simulink model "automode_simple"  (R2020b)
settings: Solver=VariableStepAuto  StartTime=0.0  StopTime=0.1  FixedStep=0.001  RelTol=1e-3
InitFcn:
  | Lf = 0.6*10^-3;
  | Cf = 1338 * 10^-6;
  | Rf = 0.019;
  | f_ac = 60;
  | f_sample = 20*10^3;
  | 
  | R_f = 19e-3;
  | L_f = 0.6e-3;
  | C_f = 1338e-6;
  | RL=2;
  | 
  | A = [0 1/C_f; -1/L_f -R_f/L_f];
  | B = [0 -1/C_f; 1/L_f 0];
  | C = [1 0; 1/RL 0; 0 1];
  | D = zeros(3,2);
libraries: fl_lib x22, nesl_utility x18, ee_lib x15, simulink x4, powerlib_meascontrol x1
settings Model: Creator=Kerim  LastModifiedBy=Kerim
settings SolverCC: ZeroCrossAlgorithm=Adaptive
settings DebuggingCC: IgnoredZcDiagnostic=none

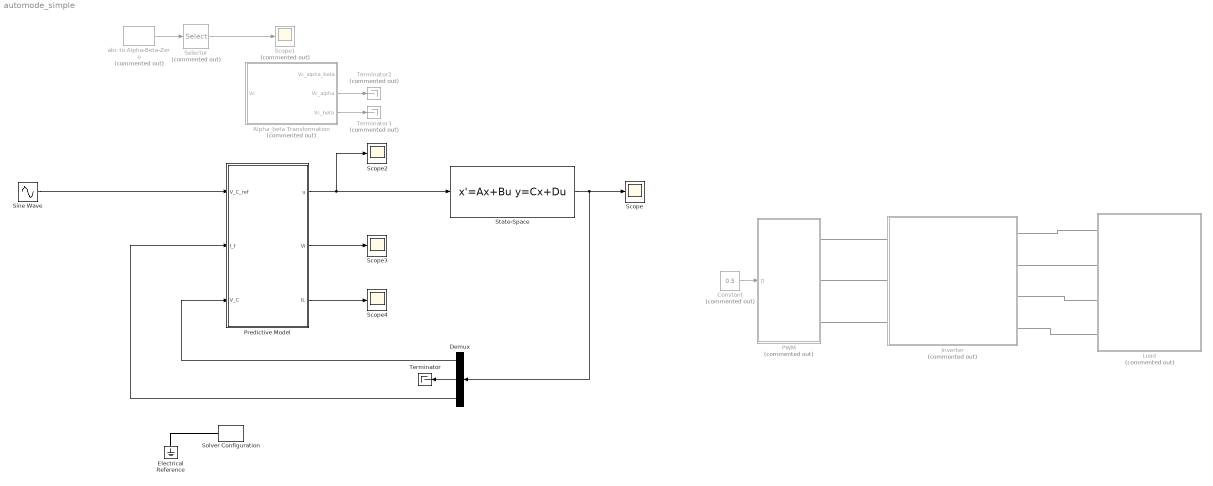
== system automode_simple ==
  Alpha_beta Transformation : MATLAB Function  Commented=on  TreatAsAtomicUnit=on
  Constant : Constant  Commented=on  Value=0.5
  Demux : Demux  Outputs=3
  Electrical Reference : fl_lib/Electrical/Electrical Elements/Electrical Reference
  Inverter : Subsystem  Commented=on
  Load : Subsystem  Commented=on
  PWM : Subsystem  Commented=on
  Predictive Model : MATLAB Function  TreatAsAtomicUnit=on  SystemSampleTime=0.001
  Scope{,2..4} (4 alike) : Scope
  Scope1 : Scope  Commented=on
  Selector : Selector  Commented=on  InputPortWidth=3  IndexOptions=Index vector (dialog)  Indices=[1 2]  OutputSizes=1
  Sine Wave : Sin  Amplitude=100  Frequency=f_ac * 2*pi  SampleTime=0
  Solver Configuration : nesl_utility/Solver Configuration  PhysicalDomain=network_engine_domain  SubClassName=solver  LeftPortType=input  RightPortType=generic  Tones=[]  Harmonics=[]  SimulateNoise=off  Profile=off  UseLocalSampling=off  EnableSwitchedLinearOptims=on  FrequencyDomain=off  UseCCode=off  RelTol=0.001  AbsTol=1e-06  MinStep=1e-09  ToWorkspace=off  RevertToSquareIcSolve=off  NumHomotopyIterations=100  PhasorMode=off  PhasorModeNumHarmonics=1  DoDC=off  ResidualTolerance=1e-9  UseLocalSolver=off  LocalSolverChoice=NE_BACKWARD_EULER_ADVANCER  LocalSolverSampleTime=1e-7  DoFixedCost=off  MaxNonlinIter=12  MaxModeIter=2  ComputeImpulses=off  ImpulseIterations=2  LinearAlgebra=auto  EquationFormulation=NE_TIME_EF  DelaysMemoryBudget=1024  AutomaticFiltering=on  FilteringTimeConstant=0.001  PartitionStorageMethod=AS_NEEDED  PartitionMemoryBudget=1024  PartitionMethod=FAST
      settings: SourceProductName=Utilities
  State-Space : StateSpace  A=A  B=B  C=C  D=D  InitialCondition=0
  Terminator : Terminator
  Terminator2 : Terminator  Commented=on
  Terminator3 : Terminator  Commented=on
  abc to Alpha-Beta-Zero : powerlib_meascontrol/Transformations/abc to Alpha-Beta-Zero  Commented=on
  wires:
  Sine Wave/1 -> Predictive Model/1(V_C_ref)
  abc to Alpha-Beta-Zero/1 -> Selector/1
  Selector/1 -> Scope1/1
  Alpha_beta Transformation/2(Vc_alpha) -> Terminator2/1
  Alpha_beta Transformation/3(Vc_beta) -> Terminator3/1
  Constant/1 -> PWM/1(D)
  Predictive Model/1(u) -> Scope2/1, State-Space/1
  Predictive Model/2(Vi) -> Scope3/1
  Predictive Model/3(IL) -> Scope4/1
  State-Space/1 -> Scope/1, Demux/1
  Demux/1 -> Predictive Model/3(V_C)
  Demux/3 -> Predictive Model/2(I_f)
  Demux/2 -> Terminator/1
  connections:
  Solver Configuration/RConn1 -- Electrical Reference/LConn1
  Load/LConn1 -- Inverter/RConn1
  Inverter/RConn2 -- Load/LConn2
  Load/LConn3 -- Inverter/RConn3
  Load/LConn4 -- Inverter/RConn4
  Inverter/LConn1 -- PWM/RConn1
  Inverter/LConn2 -- PWM/RConn2
  Inverter/LConn3 -- PWM/RConn3

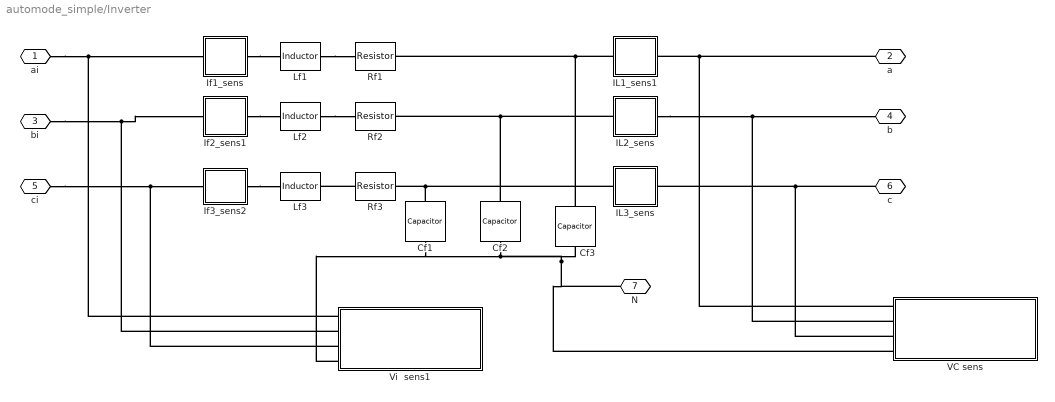
== system automode_simple/Inverter ==
  Cf1 : ee_lib/Passive/Capacitor  cap_option=0  c=Cf F  Cvec=[1e-05, 1e-06] F  Vvec=[0, 10] V  CV_table_symmetry=1  f_vec=[1, 10] kHz  DFext_vec=[.8, 1.2]  C_tol=5  enable_C_tol=0  tol_distribution=1  nSigma=4  r=1e-6 Ohm  g=0 1/Ohm  averaging_period=0 s  enable_operating_limits=0  operating_limit_action=2  max_working_voltage_range=[-25, 25] V  power_rating=1 W  enable_faults=0  fault_action=1  Cscale_faulted=100  R_faulted=1e-3 Ohm  G_faulted=0 1/Ohm  tau_fault=1e-3 s  enable_temporal_fault=0  t_fault=1 s  enable_behavioral_fault=0  max_permissible_voltage_range=[-100, 100] V  t_fail_on_voltage=1 s  i_specify=off  i_priority=None  i=0 A  i_nominal_specify=off  i_nominal_unit=A  i_nominal_value=1  v_specify=off  v_priority=None  v=0 V  v_nominal_specify=off  v_nominal_unit=V  v_nominal_value=1  vc_specify=off  vc_priority=High  vc=0 V  vc_nominal_specify=off  vc_nominal_unit=V  vc_nominal_value=1
  Cf2 : ee_lib/Passive/Capacitor  cap_option=0  c=Cf F  Cvec=[1e-05, 1e-06] F  Vvec=[0, 10] V  CV_table_symmetry=1  f_vec=[1, 10] kHz  DFext_vec=[.8, 1.2]  C_tol=5  enable_C_tol=0  tol_distribution=1  nSigma=4  r=1e-6 Ohm  g=0 1/Ohm  averaging_period=0 s  enable_operating_limits=0  operating_limit_action=2  max_working_voltage_range=[-25, 25] V  power_rating=1 W  enable_faults=0  fault_action=1  Cscale_faulted=100  R_faulted=1e-3 Ohm  G_faulted=0 1/Ohm  tau_fault=1e-3 s  enable_temporal_fault=0  t_fault=1 s  enable_behavioral_fault=0  max_permissible_voltage_range=[-100, 100] V  t_fail_on_voltage=1 s  i_specify=off  i_priority=None  i=0 A  i_nominal_specify=off  i_nominal_unit=A  i_nominal_value=1  v_specify=off  v_priority=None  v=0 V  v_nominal_specify=off  v_nominal_unit=V  v_nominal_value=1  vc_specify=off  vc_priority=High  vc=0 V  vc_nominal_specify=off  vc_nominal_unit=V  vc_nominal_value=1
  Cf3 : ee_lib/Passive/Capacitor  cap_option=0  c=Cf F  Cvec=[1e-05, 1e-06] F  Vvec=[0, 10] V  CV_table_symmetry=1  f_vec=[1, 10] kHz  DFext_vec=[.8, 1.2]  C_tol=5  enable_C_tol=0  tol_distribution=1  nSigma=4  r=1e-6 Ohm  g=0 1/Ohm  averaging_period=0 s  enable_operating_limits=0  operating_limit_action=2  max_working_voltage_range=[-25, 25] V  power_rating=1 W  enable_faults=0  fault_action=1  Cscale_faulted=100  R_faulted=1e-3 Ohm  G_faulted=0 1/Ohm  tau_fault=1e-3 s  enable_temporal_fault=0  t_fault=1 s  enable_behavioral_fault=0  max_permissible_voltage_range=[-100, 100] V  t_fail_on_voltage=1 s  i_specify=off  i_priority=None  i=0 A  i_nominal_specify=off  i_nominal_unit=A  i_nominal_value=1  v_specify=off  v_priority=None  v=0 V  v_nominal_specify=off  v_nominal_unit=V  v_nominal_value=1  vc_specify=off  vc_priority=High  vc=0 V  vc_nominal_specify=off  vc_nominal_unit=V  vc_nominal_value=1
  IL1_sens1 : Subsystem
  IL2_sens : Subsystem
  IL3_sens : Subsystem
  If1_sens : Subsystem
  If2_sens1 : Subsystem
  If3_sens2 : Subsystem
  Lf1 : ee_lib/Passive/Inductor  l=Lf H  L_tol=20  enable_L_tol=0  tol_distribution=1  nSigma=4  r=0 Ohm  g=1e-9 1/Ohm  enable_operating_limits=0  operating_limit_action=2  max_working_current=1 A  power_rating=1 W  enable_faults=0  fault_action=1  lambdaPercent=50  k_faulted=0.9999  turnsShort=0  openCct=0  groundShort=0  groundShortG=0 1/Ohm  tau_fault=1e-3 s  enable_temporal_fault=0  t_fault=1 s  enable_behavioral_fault=0  max_permissible_voltage=100 V  n_fail_on_voltage=1  max_permissible_current=1 A  t_fail_on_current=1 s  i_L_specify=off  i_L_priority=High  i_L=0 A  i_L_nominal_specify=off  i_L_nominal_unit=A  i_L_nominal_value=1
  Lf2 : ee_lib/Passive/Inductor  l=Lf H  L_tol=20  enable_L_tol=0  tol_distribution=1  nSigma=4  r=0 Ohm  g=1e-9 1/Ohm  enable_operating_limits=0  operating_limit_action=2  max_working_current=1 A  power_rating=1 W  enable_faults=0  fault_action=1  lambdaPercent=50  k_faulted=0.9999  turnsShort=0  openCct=0  groundShort=0  groundShortG=0 1/Ohm  tau_fault=1e-3 s  enable_temporal_fault=0  t_fault=1 s  enable_behavioral_fault=0  max_permissible_voltage=100 V  n_fail_on_voltage=1  max_permissible_current=1 A  t_fail_on_current=1 s  i_L_specify=off  i_L_priority=High  i_L=0 A  i_L_nominal_specify=off  i_L_nominal_unit=A  i_L_nominal_value=1
  Lf3 : ee_lib/Passive/Inductor  l=Lf H  L_tol=20  enable_L_tol=0  tol_distribution=1  nSigma=4  r=0 Ohm  g=1e-9 1/Ohm  enable_operating_limits=0  operating_limit_action=2  max_working_current=1 A  power_rating=1 W  enable_faults=0  fault_action=1  lambdaPercent=50  k_faulted=0.9999  turnsShort=0  openCct=0  groundShort=0  groundShortG=0 1/Ohm  tau_fault=1e-3 s  enable_temporal_fault=0  t_fault=1 s  enable_behavioral_fault=0  max_permissible_voltage=100 V  n_fail_on_voltage=1  max_permissible_current=1 A  t_fail_on_current=1 s  i_L_specify=off  i_L_priority=High  i_L=0 A  i_L_nominal_specify=off  i_L_nominal_unit=A  i_L_nominal_value=1
  Rf1 : ee_lib/Passive/Resistor  R=Rf Ohm  R_tol=5  enable_R_tol=0  tol_distribution=1  nSigma=4  enable_operating_limits=0  operating_limit_action=2  max_working_voltage=100 V  power_rating=1 W  enable_faults=0  fault_action=1  R_faulted=inf Ohm  enable_temporal_fault=0  t_fault=1 s  enable_behavioral_fault=0  max_permissible_current=1 A  t_fail_on_current=1 s  noise_mode=0  sample_time=1e-3 s  repeatability=1  auto_seed=3032444857  user_seed=0  Tdevice=25 degC  alpha=3.93e-3 1/K  Tmeas=25 degC  thermal_mass=100 J/K  power_derating_T1=70 degC  power_derating_T2=155 degC  operating_temperature_range_vec=[-50, 150] degC  temperature_specify=off  temperature_priority=High  temperature=298.15 K  temperature_nominal_specify=off  temperature_nominal_unit=K  temperature_nominal_value=1
  Rf2 : ee_lib/Passive/Resistor  R=Rf Ohm  R_tol=5  enable_R_tol=0  tol_distribution=1  nSigma=4  enable_operating_limits=0  operating_limit_action=2  max_working_voltage=100 V  power_rating=1 W  enable_faults=0  fault_action=1  R_faulted=inf Ohm  enable_temporal_fault=0  t_fault=1 s  enable_behavioral_fault=0  max_permissible_current=1 A  t_fail_on_current=1 s  noise_mode=0  sample_time=1e-3 s  repeatability=1  auto_seed=136721035  user_seed=0  Tdevice=25 degC  alpha=3.93e-3 1/K  Tmeas=25 degC  thermal_mass=100 J/K  power_derating_T1=70 degC  power_derating_T2=155 degC  operating_temperature_range_vec=[-50, 150] degC  temperature_specify=off  temperature_priority=High  temperature=298.15 K  temperature_nominal_specify=off  temperature_nominal_unit=K  temperature_nominal_value=1
  Rf3 : ee_lib/Passive/Resistor  R=Rf Ohm  R_tol=5  enable_R_tol=0  tol_distribution=1  nSigma=4  enable_operating_limits=0  operating_limit_action=2  max_working_voltage=100 V  power_rating=1 W  enable_faults=0  fault_action=1  R_faulted=inf Ohm  enable_temporal_fault=0  t_fault=1 s  enable_behavioral_fault=0  max_permissible_current=1 A  t_fail_on_current=1 s  noise_mode=0  sample_time=1e-3 s  repeatability=1  auto_seed=1189375164  user_seed=0  Tdevice=25 degC  alpha=3.93e-3 1/K  Tmeas=25 degC  thermal_mass=100 J/K  power_derating_T1=70 degC  power_derating_T2=155 degC  operating_temperature_range_vec=[-50, 150] degC  temperature_specify=off  temperature_priority=High  temperature=298.15 K  temperature_nominal_specify=off  temperature_nominal_unit=K  temperature_nominal_value=1
  VC sens : Subsystem
  Vi  sens1 : Subsystem
  ai : PMIOPort  Side=Left
  a : PMIOPort  Port=2  Side=Right
  bi : PMIOPort  Port=3  Side=Left
  b : PMIOPort  Port=4  Side=Right
  ci : PMIOPort  Port=5  Side=Left
  c : PMIOPort  Port=6  Side=Right
  N : PMIOPort  Port=7  Side=Right
  connections:
  Lf2/RConn1 -- Rf2/LConn1
  Lf1/RConn1 -- Rf1/LConn1
  Rf3/LConn1 -- Lf3/RConn1
  Cf2/RConn1 -- N/RConn1 -- VC sens/LConn4 -- Cf3/RConn1 -- Vi  sens1/LConn4 -- Cf1/RConn1
  c/RConn1 -- VC sens/LConn3 -- IL3_sens/RConn1
  Cf1/LConn1 -- Rf3/RConn1 -- IL3_sens/LConn1
  Cf3/LConn1 -- Rf1/RConn1 -- IL1_sens1/LConn1
  If2_sens1/RConn1 -- Lf2/LConn1
  IL2_sens/RConn1 -- VC sens/LConn2 -- b/RConn1
  Cf2/LConn1 -- Rf2/RConn1 -- IL2_sens/LConn1
  If3_sens2/RConn1 -- Lf3/LConn1
  Vi  sens1/LConn2 -- bi/RConn1 -- If2_sens1/LConn1
  a/RConn1 -- VC sens/LConn1 -- IL1_sens1/RConn1
  Vi  sens1/LConn3 -- ci/RConn1 -- If3_sens2/LConn1
  Vi  sens1/LConn1 -- ai/RConn1 -- If1_sens/LConn1
  If1_sens/RConn1 -- Lf1/LConn1

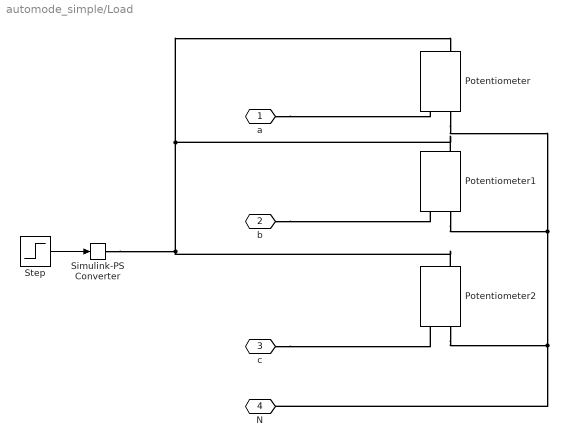
== system automode_simple/Load ==
  Potentiometer : ee_lib/Passive/Potentiometer  R0=2.16 Ohm  Rw=0.1 Ohm  Rcenter=200 Ohm  xmin=0  xmax=1  Taper=1  Gradient=1
      settings: SourceProductBaseCode=PS  InternalSimscapePortConfiguration="{\"Bottom\":[],\"Left\":[{\"id\":\"pinL\",\"label\":\"L\",\"type\":\"foundation.electrical.electrical\"},{\"id\":\"W\",\"label\":\"W\",\"type\":\"foundation.electrical.electrical\"}],\"Right\":[{\"id\":\"pinR\",\"label\":\"R\",\"type\":\"foundation.electrical.electrical\"},{\"id\":\"x\",\"label\":\"x\",\"type\":\"input\"}],\"Top\":[]}"
  Potentiometer1 : ee_lib/Passive/Potentiometer  R0=2.16 Ohm  Rw=0.1 Ohm  Rcenter=200 Ohm  xmin=0  xmax=1  Taper=1  Gradient=1
      settings: SourceProductBaseCode=PS  InternalSimscapePortConfiguration="{\"Bottom\":[],\"Left\":[{\"id\":\"pinL\",\"label\":\"L\",\"type\":\"foundation.electrical.electrical\"},{\"id\":\"W\",\"label\":\"W\",\"type\":\"foundation.electrical.electrical\"}],\"Right\":[{\"id\":\"pinR\",\"label\":\"R\",\"type\":\"foundation.electrical.electrical\"},{\"id\":\"x\",\"label\":\"x\",\"type\":\"input\"}],\"Top\":[]}"
  Potentiometer2 : ee_lib/Passive/Potentiometer  R0=2.16 Ohm  Rw=0.1 Ohm  Rcenter=200 Ohm  xmin=0  xmax=1  Taper=1  Gradient=1
      settings: SourceProductBaseCode=PS  InternalSimscapePortConfiguration="{\"Bottom\":[],\"Left\":[{\"id\":\"pinL\",\"label\":\"L\",\"type\":\"foundation.electrical.electrical\"},{\"id\":\"W\",\"label\":\"W\",\"type\":\"foundation.electrical.electrical\"}],\"Right\":[{\"id\":\"pinR\",\"label\":\"R\",\"type\":\"foundation.electrical.electrical\"},{\"id\":\"x\",\"label\":\"x\",\"type\":\"input\"}],\"Top\":[]}"
  Simulink-PS Converter : nesl_utility/Simulink-PS Converter  PhysicalDomain=network_engine_domain  SubClassName=ps_input  LeftPortType=input  RightPortType=output  PseudoPeriodic=off  Frequencies=[]  NoiseDistribution=none  NoiseParameters=[]  Unit=1  AffineConversion=off  FilteringAndDerivatives=provide  SimscapeFilterOrder=1  InputFilterTimeConstant=0.001  UdotUserProvided=0
  Step : Step  Time=0.05  Before=1  After=0.5  SampleTime=0
  a : PMIOPort  Side=Left
  b : PMIOPort  Port=2  Side=Left
  c : PMIOPort  Port=3  Side=Left
  N : PMIOPort  Port=4  Side=Left
  wires:
  Step/1 -> Simulink-PS Converter/1
  connections:
  a/RConn1 -- Potentiometer/LConn1
  b/RConn1 -- Potentiometer1/LConn1
  c/RConn1 -- Potentiometer2/LConn1
  Potentiometer/LConn2 -- Potentiometer1/LConn2 -- Potentiometer2/LConn2 -- N/RConn1
  Simulink-PS Converter/RConn1 -- Potentiometer2/RConn2 -- Potentiometer1/RConn2 -- Potentiometer/RConn2

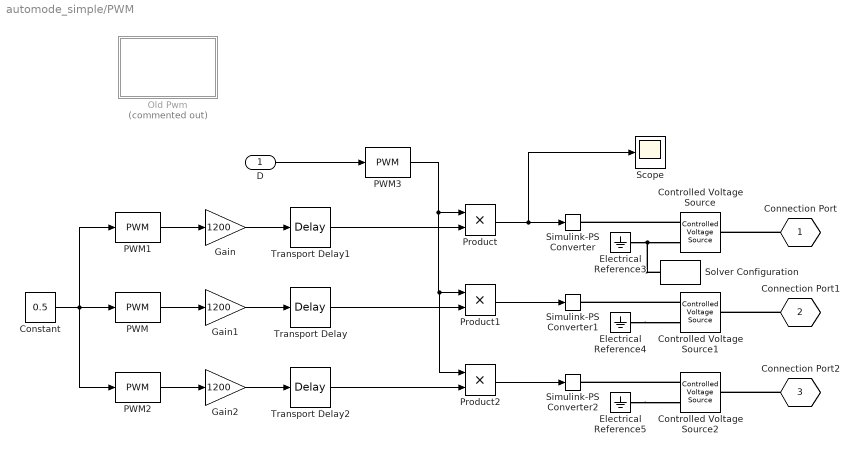
== system automode_simple/PWM ==
  D : Inport
  Constant : Constant  Value=0.5
  Controlled Voltage Source : fl_lib/Electrical/Electrical Sources/Controlled Voltage Source
  Controlled Voltage Source1 : fl_lib/Electrical/Electrical Sources/Controlled Voltage Source
  Controlled Voltage Source2 : fl_lib/Electrical/Electrical Sources/Controlled Voltage Source
  Electrical Reference3 : fl_lib/Electrical/Electrical Elements/Electrical Reference
  Electrical Reference4 : fl_lib/Electrical/Electrical Elements/Electrical Reference
  Electrical Reference5 : fl_lib/Electrical/Electrical Elements/Electrical Reference
  Gain : Gain  Gain=1200
  Gain1 : Gain  Gain=1200
  Gain2 : Gain  Gain=1200
  Old Pwm : Subsystem  Commented=on
  PWM : simulink/Discontinuities/PWM  DisableCoverage=on  Period=1/f_ac  DisallowZeroDutyCycle=off  RunAtFixedTimeIntervals=off  SampleTime=0.1
  PWM1 : simulink/Discontinuities/PWM  DisableCoverage=on  Period=1/f_ac  DisallowZeroDutyCycle=off  RunAtFixedTimeIntervals=off  SampleTime=0.1
  PWM2 : simulink/Discontinuities/PWM  DisableCoverage=on  Period=1/f_ac  DisallowZeroDutyCycle=off  RunAtFixedTimeIntervals=off  SampleTime=0.1
  PWM3 : simulink/Discontinuities/PWM  DisableCoverage=on  Period=1/f_sample  DisallowZeroDutyCycle=off  RunAtFixedTimeIntervals=off  SampleTime=0.1
  Product : Product
  Product1 : Product
  Product2 : Product
  Scope : Scope
  Simulink-PS Converter : nesl_utility/Simulink-PS Converter  PhysicalDomain=network_engine_domain  SubClassName=ps_input  LeftPortType=input  RightPortType=output  PseudoPeriodic=off  Frequencies=[]  NoiseDistribution=none  NoiseParameters=[]  Unit=1  AffineConversion=off  FilteringAndDerivatives=provide  SimscapeFilterOrder=1  InputFilterTimeConstant=0.001  UdotUserProvided=0
  Simulink-PS Converter1 : nesl_utility/Simulink-PS Converter  PhysicalDomain=network_engine_domain  SubClassName=ps_input  LeftPortType=input  RightPortType=output  PseudoPeriodic=off  Frequencies=[]  NoiseDistribution=none  NoiseParameters=[]  Unit=1  AffineConversion=off  FilteringAndDerivatives=provide  SimscapeFilterOrder=1  InputFilterTimeConstant=0.001  UdotUserProvided=0
  Simulink-PS Converter2 : nesl_utility/Simulink-PS Converter  PhysicalDomain=network_engine_domain  SubClassName=ps_input  LeftPortType=input  RightPortType=output  PseudoPeriodic=off  Frequencies=[]  NoiseDistribution=none  NoiseParameters=[]  Unit=1  AffineConversion=off  FilteringAndDerivatives=provide  SimscapeFilterOrder=1  InputFilterTimeConstant=0.001  UdotUserProvided=0
  Solver Configuration : nesl_utility/Solver Configuration  PhysicalDomain=network_engine_domain  SubClassName=solver  LeftPortType=input  RightPortType=generic  Tones=[]  Harmonics=[]  SimulateNoise=off  Profile=off  UseLocalSampling=off  EnableSwitchedLinearOptims=on  FrequencyDomain=off  UseCCode=off  RelTol=0.001  AbsTol=1e-06  MinStep=1e-09  ToWorkspace=off  RevertToSquareIcSolve=off  NumHomotopyIterations=100  PhasorMode=off  PhasorModeNumHarmonics=1  DoDC=off  ResidualTolerance=1e-9  UseLocalSolver=off  LocalSolverChoice=NE_BACKWARD_EULER_ADVANCER  LocalSolverSampleTime=1e-7  DoFixedCost=off  MaxNonlinIter=12  MaxModeIter=2  ComputeImpulses=off  ImpulseIterations=2  LinearAlgebra=auto  EquationFormulation=NE_TIME_EF  DelaysMemoryBudget=1024  AutomaticFiltering=on  FilteringTimeConstant=0.001  PartitionStorageMethod=AS_NEEDED  PartitionMemoryBudget=1024  PartitionMethod=FAST
      settings: SourceProductName=Utilities
  Transport Delay : TransportDelay  DelayTime=(1/f_ac)/3
  Transport Delay1 : TransportDelay  DelayTime=0
  Transport Delay2 : TransportDelay  DelayTime=2*(1/f_ac)/3
  Connection Port : PMIOPort  Tag=PMCPort  Side=Right
  Connection Port1 : PMIOPort  Tag=PMCPort  Port=2  Side=Right
  Connection Port2 : PMIOPort  Tag=PMCPort  Port=3  Side=Right
  wires:
  Constant/1 -> PWM2/1, PWM1/1, PWM/1
  Transport Delay/1 -> Product1/2
  Transport Delay2/1 -> Product2/2
  PWM1/1 -> Gain/1
  Gain/1 -> Transport Delay1/1
  PWM/1 -> Gain1/1
  Gain1/1 -> Transport Delay/1
  Gain2/1 -> Transport Delay2/1
  PWM2/1 -> Gain2/1
  PWM3/1 -> Product/1, Product2/1, Product1/1
  Transport Delay1/1 -> Product/2
  D/1 -> PWM3/1
  Product/1 -> Scope/1, Simulink-PS Converter/1
  Product1/1 -> Simulink-PS Converter1/1
  Product2/1 -> Simulink-PS Converter2/1
  connections:
  Controlled Voltage Source/RConn1 -- Simulink-PS Converter/RConn1
  Electrical Reference3/LConn1 -- Solver Configuration/RConn1 -- Controlled Voltage Source/RConn2
  Electrical Reference4/LConn1 -- Controlled Voltage Source1/RConn2
  Controlled Voltage Source1/RConn1 -- Simulink-PS Converter1/RConn1
  Electrical Reference5/LConn1 -- Controlled Voltage Source2/RConn2
  Controlled Voltage Source2/RConn1 -- Simulink-PS Converter2/RConn1
  Connection Port/RConn1 -- Controlled Voltage Source/LConn1
  Connection Port1/RConn1 -- Controlled Voltage Source1/LConn1
  Connection Port2/RConn1 -- Controlled Voltage Source2/LConn1

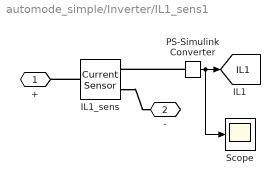
== system automode_simple/Inverter/IL1_sens1 ==
  IL1_sens : fl_lib/Electrical/Electrical Sensors/Current Sensor
  PS-Simulink Converter : nesl_utility/PS-Simulink Converter  PhysicalDomain=network_engine_domain  SubClassName=ps_output  LeftPortType=input  RightPortType=output  PseudoPeriodic=off  Frequencies=[]  Unit=inherit  AffineConversion=off
  Scope : Scope
  + : PMIOPort  Side=Left
  - : PMIOPort  Port=2  Side=Right
  tag scope: IL1=global
  wires:
  PS-Simulink Converter/1 -> Scope/1, [IL1]
  connections:
  IL1_sens/RConn2 -- -/RConn1
  IL1_sens/LConn1 -- +/RConn1
  PS-Simulink Converter/LConn1 -- IL1_sens/RConn1

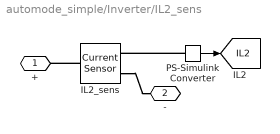
== system automode_simple/Inverter/IL2_sens ==
  IL2_sens : fl_lib/Electrical/Electrical Sensors/Current Sensor
  PS-Simulink Converter : nesl_utility/PS-Simulink Converter  PhysicalDomain=network_engine_domain  SubClassName=ps_output  LeftPortType=input  RightPortType=output  PseudoPeriodic=off  Frequencies=[]  Unit=inherit  AffineConversion=off
  + : PMIOPort  Side=Left
  - : PMIOPort  Port=2  Side=Right
  tag scope: IL2=global
  wires:
  PS-Simulink Converter/1 -> [IL2]
  connections:
  IL2_sens/RConn2 -- -/RConn1
  IL2_sens/LConn1 -- +/RConn1
  PS-Simulink Converter/LConn1 -- IL2_sens/RConn1

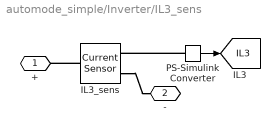
== system automode_simple/Inverter/IL3_sens ==
  IL3_sens : fl_lib/Electrical/Electrical Sensors/Current Sensor
  PS-Simulink Converter : nesl_utility/PS-Simulink Converter  PhysicalDomain=network_engine_domain  SubClassName=ps_output  LeftPortType=input  RightPortType=output  PseudoPeriodic=off  Frequencies=[]  Unit=inherit  AffineConversion=off
  + : PMIOPort  Side=Left
  - : PMIOPort  Port=2  Side=Right
  tag scope: IL3=global
  wires:
  PS-Simulink Converter/1 -> [IL3]
  connections:
  IL3_sens/RConn2 -- -/RConn1
  IL3_sens/LConn1 -- +/RConn1
  PS-Simulink Converter/LConn1 -- IL3_sens/RConn1

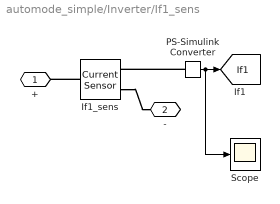
== system automode_simple/Inverter/If1_sens ==
  If1_sens : fl_lib/Electrical/Electrical Sensors/Current Sensor
  PS-Simulink Converter : nesl_utility/PS-Simulink Converter  PhysicalDomain=network_engine_domain  SubClassName=ps_output  LeftPortType=input  RightPortType=output  PseudoPeriodic=off  Frequencies=[]  Unit=inherit  AffineConversion=off
  Scope : Scope
  + : PMIOPort  Side=Left
  - : PMIOPort  Port=2  Side=Right
  tag scope: If1=global
  wires:
  PS-Simulink Converter/1 -> Scope/1, [If1]
  connections:
  If1_sens/RConn2 -- -/RConn1
  If1_sens/LConn1 -- +/RConn1
  PS-Simulink Converter/LConn1 -- If1_sens/RConn1

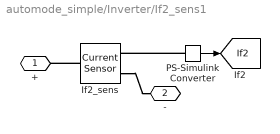
== system automode_simple/Inverter/If2_sens1 ==
  If2_sens : fl_lib/Electrical/Electrical Sensors/Current Sensor
  PS-Simulink Converter : nesl_utility/PS-Simulink Converter  PhysicalDomain=network_engine_domain  SubClassName=ps_output  LeftPortType=input  RightPortType=output  PseudoPeriodic=off  Frequencies=[]  Unit=inherit  AffineConversion=off
  + : PMIOPort  Side=Left
  - : PMIOPort  Port=2  Side=Right
  tag scope: If2=global
  wires:
  PS-Simulink Converter/1 -> [If2]
  connections:
  If2_sens/RConn2 -- -/RConn1
  If2_sens/LConn1 -- +/RConn1
  PS-Simulink Converter/LConn1 -- If2_sens/RConn1

== system automode_simple/Inverter/If3_sens2 ==
  If1_sens : fl_lib/Electrical/Electrical Sensors/Current Sensor
  PS-Simulink Converter : nesl_utility/PS-Simulink Converter  PhysicalDomain=network_engine_domain  SubClassName=ps_output  LeftPortType=input  RightPortType=output  PseudoPeriodic=off  Frequencies=[]  Unit=inherit  AffineConversion=off
  + : PMIOPort  Side=Left
  - : PMIOPort  Port=2  Side=Right
  tag scope: If3=global
  wires:
  PS-Simulink Converter/1 -> [If3]
  connections:
  If1_sens/RConn2 -- -/RConn1
  If1_sens/LConn1 -- +/RConn1
  PS-Simulink Converter/LConn1 -- If1_sens/RConn1

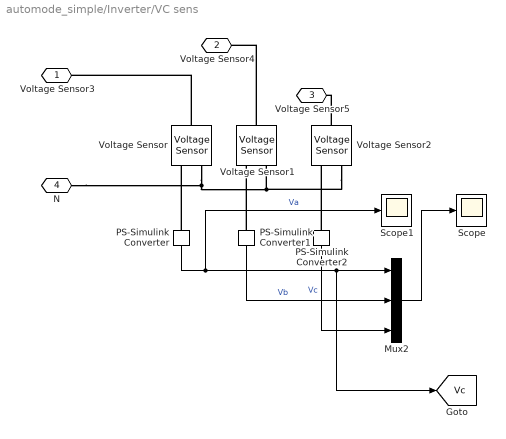
== system automode_simple/Inverter/VC sens ==
  Mux2 : Mux  Inputs=3
  PS-Simulink Converter : nesl_utility/PS-Simulink Converter  PhysicalDomain=network_engine_domain  SubClassName=ps_output  LeftPortType=input  RightPortType=output  PseudoPeriodic=off  Frequencies=[]  Unit=inherit  AffineConversion=off
  PS-Simulink Converter1 : nesl_utility/PS-Simulink Converter  PhysicalDomain=network_engine_domain  SubClassName=ps_output  LeftPortType=input  RightPortType=output  PseudoPeriodic=off  Frequencies=[]  Unit=inherit  AffineConversion=off
  PS-Simulink Converter2 : nesl_utility/PS-Simulink Converter  PhysicalDomain=network_engine_domain  SubClassName=ps_output  LeftPortType=input  RightPortType=output  PseudoPeriodic=off  Frequencies=[]  Unit=inherit  AffineConversion=off
  Scope : Scope
  Scope1 : Scope
  Voltage Sensor : fl_lib/Electrical/Electrical Sensors/Voltage Sensor
  Voltage Sensor1 : fl_lib/Electrical/Electrical Sensors/Voltage Sensor
  Voltage Sensor2 : fl_lib/Electrical/Electrical Sensors/Voltage Sensor
  Voltage Sensor3 : PMIOPort  Side=Left
  Voltage Sensor4 : PMIOPort  Port=2  Side=Left
  Voltage Sensor5 : PMIOPort  Port=3  Side=Left
  N : PMIOPort  Port=4  Side=Left
  tag scope: Vc=global
  wires:
  PS-Simulink Converter/1 -> Scope1/1, [Vc], Mux2/1  "Va"
  PS-Simulink Converter1/1 -> Mux2/2  "Vb"
  PS-Simulink Converter2/1 -> Mux2/3  "Vc"
  Mux2/1 -> Scope/1
  connections:
  PS-Simulink Converter2/LConn1 -- Voltage Sensor2/RConn1
  Voltage Sensor/RConn2 -- N/RConn1 -- Voltage Sensor2/RConn2 -- Voltage Sensor1/RConn2
  Voltage Sensor/LConn1 -- Voltage Sensor3/RConn1
  PS-Simulink Converter/LConn1 -- Voltage Sensor/RConn1
  PS-Simulink Converter1/LConn1 -- Voltage Sensor1/RConn1
  Voltage Sensor2/LConn1 -- Voltage Sensor5/RConn1
  Voltage Sensor1/LConn1 -- Voltage Sensor4/RConn1

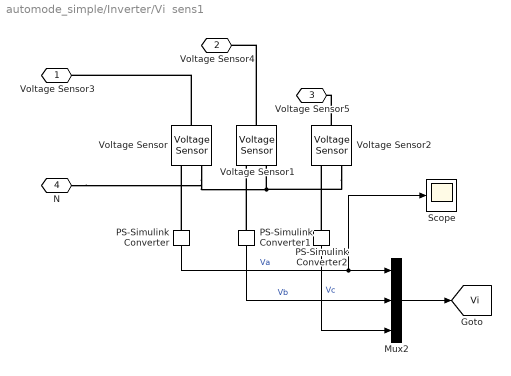
== system automode_simple/Inverter/Vi  sens1 ==
  Mux2 : Mux  Inputs=3
  PS-Simulink Converter : nesl_utility/PS-Simulink Converter  PhysicalDomain=network_engine_domain  SubClassName=ps_output  LeftPortType=input  RightPortType=output  PseudoPeriodic=off  Frequencies=[]  Unit=inherit  AffineConversion=off
  PS-Simulink Converter1 : nesl_utility/PS-Simulink Converter  PhysicalDomain=network_engine_domain  SubClassName=ps_output  LeftPortType=input  RightPortType=output  PseudoPeriodic=off  Frequencies=[]  Unit=inherit  AffineConversion=off
  PS-Simulink Converter2 : nesl_utility/PS-Simulink Converter  PhysicalDomain=network_engine_domain  SubClassName=ps_output  LeftPortType=input  RightPortType=output  PseudoPeriodic=off  Frequencies=[]  Unit=inherit  AffineConversion=off
  Scope : Scope
  Voltage Sensor : fl_lib/Electrical/Electrical Sensors/Voltage Sensor
  Voltage Sensor1 : fl_lib/Electrical/Electrical Sensors/Voltage Sensor
  Voltage Sensor2 : fl_lib/Electrical/Electrical Sensors/Voltage Sensor
  Voltage Sensor3 : PMIOPort  Side=Left
  Voltage Sensor4 : PMIOPort  Port=2  Side=Left
  Voltage Sensor5 : PMIOPort  Port=3  Side=Left
  N : PMIOPort  Port=4  Side=Left
  tag scope: Vi=global
  wires:
  PS-Simulink Converter/1 -> Scope/1, Mux2/1  "Va"
  PS-Simulink Converter1/1 -> Mux2/2  "Vb"
  PS-Simulink Converter2/1 -> Mux2/3  "Vc"
  Mux2/1 -> [Vi]
  connections:
  PS-Simulink Converter2/LConn1 -- Voltage Sensor2/RConn1
  Voltage Sensor2/RConn2 -- N/RConn1 -- Voltage Sensor/RConn2 -- Voltage Sensor1/RConn2
  Voltage Sensor/LConn1 -- Voltage Sensor3/RConn1
  PS-Simulink Converter/LConn1 -- Voltage Sensor/RConn1
  PS-Simulink Converter1/LConn1 -- Voltage Sensor1/RConn1
  Voltage Sensor2/LConn1 -- Voltage Sensor5/RConn1
  Voltage Sensor1/LConn1 -- Voltage Sensor4/RConn1

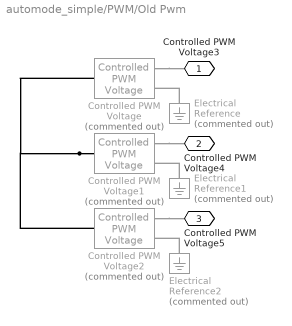
== system automode_simple/PWM/Old Pwm ==
  Controlled PWM Voltage : ee_lib/Integrated Circuits/Controlled PWM Voltage  Commented=on  F=f_ac Hz  TD=0 s  pulse_width_offset=0 s  pulse_min=0 s  Vmin=0 V  Vmax=5 V  Vm=1200 V  pwm_or_av=1  event_type=1  sample_time=1e-6 s  u_min=0  u_max=1
      settings: InternalSimscapePortConfiguration="{\"Bottom\":[],\"Left\":[{\"id\":\"u\",\"label\":\"u\",\"type\":\"input\"}],\"Right\":[{\"id\":\"p2\",\"label\":\"PWM\",\"type\":\"foundation.electrical.electrical\"},{\"id\":\"n2\",\"label\":\"REF\",\"type\":\"foundation.electrical.electrical\"}],\"Top\":[]}"
  Controlled PWM Voltage1 : ee_lib/Integrated Circuits/Controlled PWM Voltage  Commented=on  F=f_ac Hz  TD=(1/f_ac)/3 s  pulse_width_offset=0 s  pulse_min=0 s  Vmin=0 V  Vmax=5 V  Vm=1200 V  pwm_or_av=1  event_type=1  sample_time=1e-6 s  u_min=0  u_max=1
      settings: InternalSimscapePortConfiguration="{\"Bottom\":[],\"Left\":[{\"id\":\"u\",\"label\":\"u\",\"type\":\"input\"}],\"Right\":[{\"id\":\"p2\",\"label\":\"PWM\",\"type\":\"foundation.electrical.electrical\"},{\"id\":\"n2\",\"label\":\"REF\",\"type\":\"foundation.electrical.electrical\"}],\"Top\":[]}"
  Controlled PWM Voltage2 : ee_lib/Integrated Circuits/Controlled PWM Voltage  Commented=on  F=f_ac Hz  TD=2*(1/f_ac)/3 s  pulse_width_offset=0 s  pulse_min=0 s  Vmin=0 V  Vmax=5 V  Vm=1200 V  pwm_or_av=1  event_type=1  sample_time=1e-6 s  u_min=0  u_max=1
      settings: InternalSimscapePortConfiguration="{\"Bottom\":[],\"Left\":[{\"id\":\"u\",\"label\":\"u\",\"type\":\"input\"}],\"Right\":[{\"id\":\"p2\",\"label\":\"PWM\",\"type\":\"foundation.electrical.electrical\"},{\"id\":\"n2\",\"label\":\"REF\",\"type\":\"foundation.electrical.electrical\"}],\"Top\":[]}"
  Electrical Reference : fl_lib/Electrical/Electrical Elements/Electrical Reference  Commented=on
  Electrical Reference1 : fl_lib/Electrical/Electrical Elements/Electrical Reference  Commented=on
  Electrical Reference2 : fl_lib/Electrical/Electrical Elements/Electrical Reference  Commented=on
  Controlled PWM Voltage3 : PMIOPort  Side=Right
  Controlled PWM Voltage4 : PMIOPort  Port=2  Side=Right
  Controlled PWM Voltage5 : PMIOPort  Port=3  Side=Right
  connections:
  Controlled PWM Voltage/RConn1 -- Controlled PWM Voltage3/RConn1
  Electrical Reference1/LConn1 -- Controlled PWM Voltage1/RConn2
  Electrical Reference/LConn1 -- Controlled PWM Voltage/RConn2
  Electrical Reference2/LConn1 -- Controlled PWM Voltage2/RConn2
  Controlled PWM Voltage2/RConn1 -- Controlled PWM Voltage5/RConn1
  Controlled PWM Voltage1/LConn1 -- Controlled PWM Voltage2/LConn1 -- Controlled PWM Voltage/LConn1
  Controlled PWM Voltage1/RConn1 -- Controlled PWM Voltage4/RConn1

== matlab function automode_simple/Alpha_beta Transformation ==
  data: Vc_alpha_beta output; Vc input; Vc_alpha output; Vc_beta output
function [Vc_alpha_beta, Vc_alpha, Vc_beta] = fcn(Vc)

Vc_alpha_beta = 2/3 * [1 -1/2 -1/2; 0 sqrt(3)/2 -sqrt(3)/2] * Vc;
Vc_alpha = Vc_alpha_beta(1);
Vc_beta = Vc_alpha_beta(2);

== matlab function automode_simple/Predictive Model ==
  data: V_C_ref input; I_f input; V_C input; u output; Vi output; IL output
function [u, Vi, IL]  = fcn(V_C_ref, I_f, V_C)
coder.extrinsic('quadprog');
Ts  = 0.001;      % [s] 
R_f = 19e-3;     % [ohm]
L_f = 0.6e-3;    % [H]
C_f = 1338e-6;   % [F]
u = zeros(2,1); Vi = 0;
% State Space Equations for auto mode.

ub = [800 ; 400];
lb = -ub;


x = [V_C I_f]';

A = [0 1/C_f; -1/L_f -R_f/L_f];
B = [0 -1/C_f; 1/L_f 0];

% Ad = eye(2) + A * Ts;
% Bd =  A^(-1) * (Ad - eye(2)) * B;

Ad = exp(A*Ts);
Bd = A^-1 * (exp(A*Ts) - eye(2)) * B;

RL=2;


Adv = Ad(1,:); Bdv = Bd(1,:);


alpha_M = 2/3 * [1 -1/2 -1/2; 0 sqrt(3)/2 -sqrt(3)/2];
%x_kp = Ad * x  + Bd * y;
%V_C_kp = x_kp(1,:);    % Prediction value of capacitor

%x_tilda = x * alpha_M';
%u_tilda = u' * Bdv';
F = Adv; H = Bdv;
Mu = H'*H;
f  = H'*F*x-H'* V_C_ref;
u=quadprog(2*Mu,2*f,[],[],[],[],lb,ub);
Vi = u(1,:); IL = u(2,:);
%D = Vi/V_C_kp;



%% COST FUNCTION
% Vc_alpha_beta = alpha_M * V_C;
% Vc_alpha = Vc_alpha_beta(1);
% Vc_beta = Vc_alpha_beta(2);

% J_V = (V_C_alpha_ref - Vc_alpha)^2 + (V_C_beta_ref - Vc_beta)^2;
% H = 2;
% f = 0;
% 
% % ITS TEMPORARY WRITTEN
% u_a = J_V(1);
% u_b = J_V(2);
% u_c = J_V(3);

%% EOF
